simulink model "exnb4137986_Q5"  (R2023b)
settings: Solver=FixedStepAuto  StartTime=0.0  StopTime=20  FixedStep=0.01  RelTol=1e-3
values from neighbouring files (symbols this model uses):
  equ_1 = [u_star_1, x_star_1]    [exnb4137986_Q5_par.m]    (also in exnb4137986_Q6_par.m)
  equ_2 = [u_star_2, x_star_2]    [exnb4137986_Q5_par.m]    (also in exnb4137986_Q6_par.m)
  K = place(A, B, lambda_cl)    [exnb4137986_Q5_par.m]    (also in exnb4137986_Q6_par.m)
  values = [0.005, 10]    [exnb4137986_Q3_par.m]    (also in exnb4137986_Q5_par.m; exnb4137986_Q6_par.m)
settings Model: Creator=therkelsen  LastModifiedBy=therkelsen

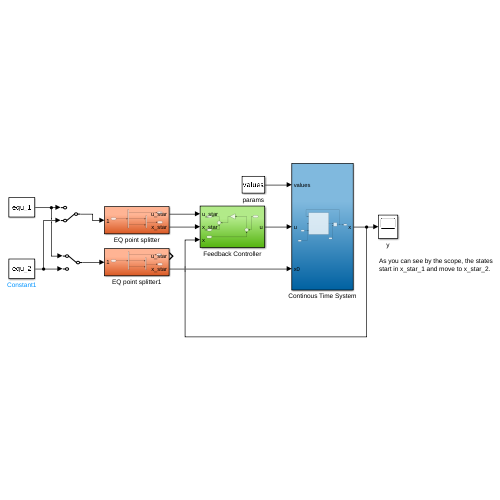
[thumbnail: Simulink's stored preview of the top-level diagram]
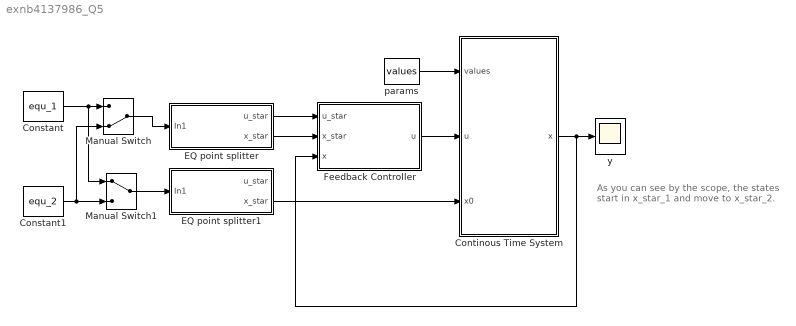
== system exnb4137986_Q5 ==
  note: As you can see by the scope, the states
      | start in x_star_1 and move to x_star_2.
  Constant : Constant  Value=equ_1
  Constant1 : Constant  Value=equ_2
  Continous Time System : Subsystem
  EQ point splitter : Subsystem
  EQ point splitter1 : Subsystem
  Feedback Controller : Subsystem
  Manual Switch : ManualSwitch  CurrentSetting=0
  Manual Switch1 : ManualSwitch
  params : Constant  Value=values
  y : Scope
  wires:
  Continous Time System/1(x) -> Feedback Controller/3(x), y/1
  Feedback Controller/1(u) -> Continous Time System/2(u)
  params/1 -> Continous Time System/1(values)
  EQ point splitter/1(u_star) -> Feedback Controller/1(u_star)
  EQ point splitter/2(x_star) -> Feedback Controller/2(x_star)
  Manual Switch/1 -> EQ point splitter/1(In1)
  Constant1/1 -> Manual Switch/2, Manual Switch1/2
  Constant/1 -> Manual Switch1/1, Manual Switch/1
  Manual Switch1/1 -> EQ point splitter1/1(In1)
  EQ point splitter1/2(x_star) -> Continous Time System/3(x0)

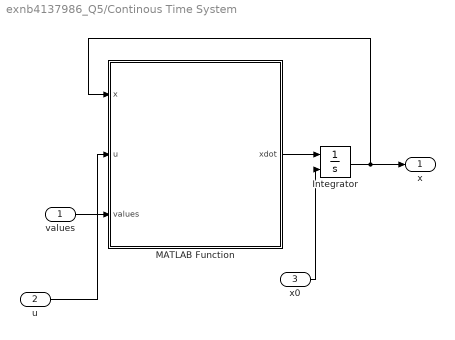
== system exnb4137986_Q5/Continous Time System ==
  values : Inport
  u : Inport  Port=2
  x0 : Inport  Port=3
  Integrator : Integrator  InitialConditionSource=external
  MATLAB Function : MATLAB Function  TreatAsAtomicUnit=on
  x : Outport
  wires:
  MATLAB Function/1(xdot) -> Integrator/1
  values/1 -> MATLAB Function/3(values)
  u/1 -> MATLAB Function/2(u)
  x0/1 -> Integrator/2
  Integrator/1 -> x/1, MATLAB Function/1(x)

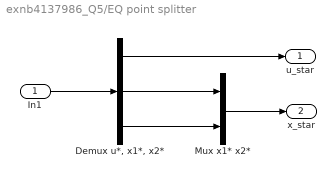
== system exnb4137986_Q5/EQ point splitter ==
  In1 : Inport
  "Demux u*, x1*, x2*" : Demux  Outputs=3
  Mux x1* x2* : Mux  Inputs=2
  u_star : Outport
  x_star : Outport  Port=2
  wires:
  "Demux u*, x1*, x2*"/3 -> Mux x1* x2*/2
  Mux x1* x2*/1 -> x_star/1
  "Demux u*, x1*, x2*"/2 -> Mux x1* x2*/1
  "Demux u*, x1*, x2*"/1 -> u_star/1
  In1/1 -> "Demux u*, x1*, x2*"/1

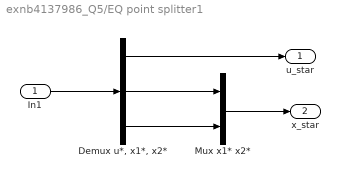
== system exnb4137986_Q5/EQ point splitter1 ==
  In1 : Inport
  "Demux u*, x1*, x2*" : Demux  Outputs=3
  Mux x1* x2* : Mux  Inputs=2
  u_star : Outport
  x_star : Outport  Port=2
  wires:
  "Demux u*, x1*, x2*"/3 -> Mux x1* x2*/2
  Mux x1* x2*/1 -> x_star/1
  "Demux u*, x1*, x2*"/2 -> Mux x1* x2*/1
  "Demux u*, x1*, x2*"/1 -> u_star/1
  In1/1 -> "Demux u*, x1*, x2*"/1

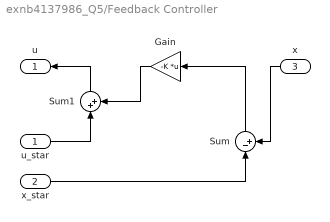
== system exnb4137986_Q5/Feedback Controller ==
  u_star : Inport
  x_star : Inport  Port=2
  x : Inport  Port=3
  Gain : Gain  Gain=-K  Multiplication=Matrix(K*u)
  Sum : Sum  Inputs=|-+
  Sum1 : Sum  Inputs=|++
  u : Outport
  wires:
  x/1 -> Sum/2
  Gain/1 -> Sum1/2
  Sum/1 -> Gain/1
  x_star/1 -> Sum/1
  u_star/1 -> Sum1/1
  Sum1/1 -> u/1

== matlab function exnb4137986_Q5/Continous Time System/MATLAB Function ==
  data: x input; u input; xdot output; values input
function xdot = fcn(x, u, values)

d = values(1);
lambda = values(2);

xdot = [-d*x(1)*abs(x(1)) + x(2);
         -lambda*x(2) + u];
